simulink model "part_b"  (R2020b)
settings: Solver=VariableStepAuto  StartTime=0.0  StopTime=0.01  FixedStep=1e-9  RelTol=1e-3
libraries: powerlib x19, powerlib_meascontrol x1
settings Model: Creator=apurv  LastModifiedBy=apurv

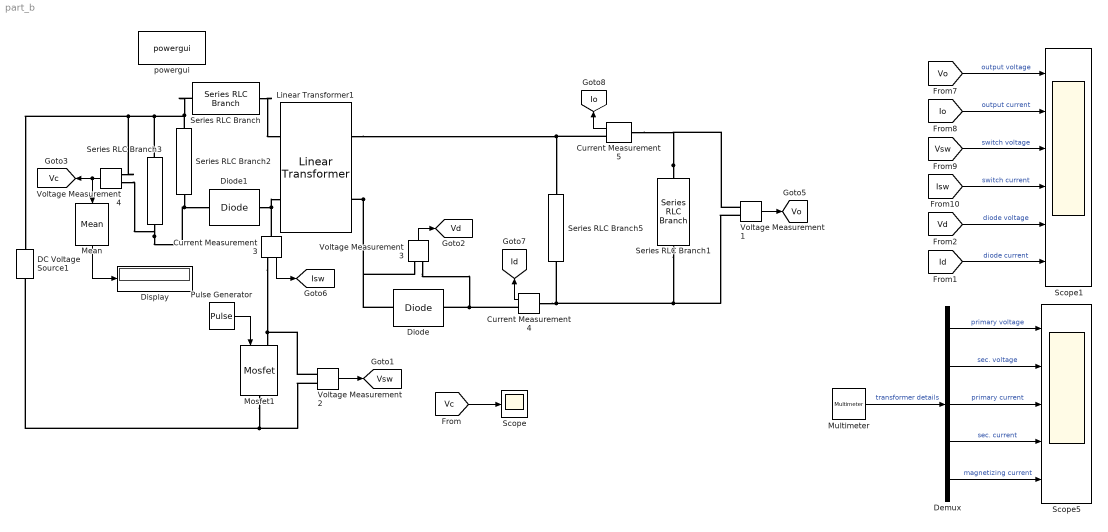
== system part_b ==
  Current Measurement3 : powerlib/Measurements/Current Measurement  PhasorSimulation=off  OutputType=Complex  PSBequivalent=0
  Current Measurement4 : powerlib/Measurements/Current Measurement  PhasorSimulation=off  OutputType=Complex  PSBequivalent=0
  Current Measurement5 : powerlib/Measurements/Current Measurement  PhasorSimulation=off  OutputType=Complex  PSBequivalent=0
  DC Voltage Source1 : powerlib/Electrical Sources/DC Voltage Source  Amplitude=24  Measurements=None
  Demux : Demux  Outputs=5
  Diode : powerlib/Power Electronics/Diode  Ron=1e-6  Lon=0  Vf=0  IC=0  UseSnubber=0  Rs=inf  Cs=0  Measurements=off
  Diode1 : powerlib/Power Electronics/Diode  Ron=1e-6  Lon=0  Vf=0  IC=0  UseSnubber=0  Rs=inf  Cs=0  Measurements=off
  Display : Display
  Linear Transformer1 : powerlib/Elements/Linear Transformer  UNITS=SI  NominalPower=[20 100000 ]  winding1=[30 0 0]  winding2=[10 0 0]  ThreeWindings=off  winding3=[3.15e+05 0.7938 0.084225]  RmLm=[1e12 250e-6]  Measurements=All voltages and currents  DataType=on
  Mean : powerlib_meascontrol/Measurements/Mean  Freq=100000  Vinit=0  Ts=0
  Mosfet1 : powerlib/Power Electronics/Mosfet  Ron=1e-6  Lon=0  Rd=1e-6  Vfd=0  IC=0  Rs=1e12  Cs=inf  Measurements=off
  Multimeter : powerlib/Measurements/Multimeter  PhasorSimulation=off  OutputType=Complex  sel=[1 2 3 4 6]  L=7  Gain=[1 1 1 1 1]  yselected={'Uw1: Linear Transformer1','Uw2: Linear Transformer1','Iw1: Linear Transformer1','Iw2: Linear Transformer1','Imag: Linear Transformer1'};  PSBOutputType=1  PSBequivalent=0  AxesSetting=[0,0.1,-100,100]  Display=0  SavedBlockNames=-11
  Pulse Generator : DiscretePulseGenerator  PulseType=Time based  Period=1/100000  PulseWidth=40
  Scope : Scope
  Scope1 : Scope  NumInputPorts=6
  Scope5 : Scope  NumInputPorts=5
  Series RLC Branch : powerlib/Elements/Series RLC Branch  LConnTagsString=__new0  RConnTagsString=__new0  BranchType=L  Resistance=1  Inductance=450e-9  SetiL0=off  InitialCurrent=0  Capacitance=1e-6  Setx0=off  InitialVoltage=0  Measurements=None
  Series RLC Branch1 : powerlib/Elements/Series RLC Branch  LConnTagsString=__new0  RConnTagsString=__new0  BranchType=R  Resistance=1  Inductance=1e-3  SetiL0=off  InitialCurrent=0  Capacitance=1e-6  Setx0=off  InitialVoltage=0  Measurements=None
  Series RLC Branch2 : powerlib/Elements/Series RLC Branch  LConnTagsString=__new0  RConnTagsString=__new0  BranchType=R  Resistance=5000  Inductance=1e-3  SetiL0=off  InitialCurrent=0  Capacitance=100e-6  Setx0=off  InitialVoltage=0  Measurements=None
  Series RLC Branch3 : powerlib/Elements/Series RLC Branch  LConnTagsString=__new0  RConnTagsString=__new0  BranchType=C  Resistance=0  Inductance=1e-3  SetiL0=off  InitialCurrent=0  Capacitance=10e-9  Setx0=off  InitialVoltage=0  Measurements=None
  Series RLC Branch5 : powerlib/Elements/Series RLC Branch  LConnTagsString=__new0  RConnTagsString=__new0  BranchType=C  Resistance=0  Inductance=1e-3  SetiL0=off  InitialCurrent=0  Capacitance=100e-6  Setx0=off  InitialVoltage=0  Measurements=None
  Voltage Measurement{1..4} (4 alike) : powerlib/Measurements/Voltage Measurement  PhasorSimulation=off  OutputType=Complex  PSBequivalent=0
  powergui : powerlib/powergui  Priority=1  SimulationMode=Discrete  SampleTime=1e-7  frequency=60  Iterations=50  frequencyindice=0  Pbase=100e6  ErrMax=1e-4  UnitsV=kV  UnitsW=MW  buscounter=0  FunctionMessages=off  echomessages=off  EnableUseOfTLC=off  CurrentSourceSwitches=off  DisableSnubberDevices=off  DisableRonSwitches=off  DisableVfSwitches=off  DisplayEquations=off  AutomaticDiscreteSolvers=off  SolverType=Tustin/Backward Euler (TBE)  Interpol=off  ExternalGateDelay=off  methode=off  Ts=100  x0status=blocks  SPID=on  SwTol=0  HookPort=off  NonlinearTolerance=1e-4  nMaxIteration=100  ContinueOnMaxIteration=off  RestoreLinks=warning  ResistiveCurrentMeasurement=off  Frange=[0:2:500]  Ylog=off  Xlog=on  ShowGrid=off  save=off  variable=ZData  structure=0  ZoomFFT=off  StartTime=0.0  cycles=1  DisplayStyle=1  fundamental=60  FreqAxis=off  MaxFrequency=1000  frequencyindicesteady=1  RmsSteady=1  display=off
  tag scope: Id=global, Io=global, Isw=global, Vc=global, Vd=global, Vo=global, Vsw=global
  wires:
  Demux/3 -> Scope5/3  "primary current"
  [Vo] -> Scope1/1  "output voltage"
  Multimeter/1 -> Demux/1  "transformer details"
  [Vd] -> Scope1/5  "diode voltage"
  Demux/5 -> Scope5/5  "magnetizing current"
  Demux/4 -> Scope5/4  "sec. current"
  Voltage Measurement2/1 -> [Vsw]
  [Io] -> Scope1/2  "output current"
  Voltage Measurement3/1 -> [Vd]
  [Id] -> Scope1/6  "diode current"
  Demux/1 -> Scope5/1  "primary voltage"
  [Isw] -> Scope1/4  "switch current"
  Current Measurement4/1 -> [Id]
  Current Measurement3/1 -> [Isw]
  [Vsw] -> Scope1/3  "switch voltage"
  Current Measurement5/1 -> [Io]
  Demux/2 -> Scope5/2  "sec. voltage"
  Voltage Measurement1/1 -> [Vo]
  Pulse Generator/1 -> Mosfet1/1
  Voltage Measurement4/1 -> Mean/1, [Vc]
  [Vc] -> Scope/1
  Mean/1 -> Display/1
  connections:
  Voltage Measurement2/LConn2 -- Mosfet1/RConn1 -- DC Voltage Source1/LConn1
  Voltage Measurement3/LConn2 -- Current Measurement4/RConn1 -- Diode/RConn1
  Linear Transformer1/RConn2 -- Diode/LConn1 -- Voltage Measurement3/LConn1
  Series RLC Branch1/LConn1 -- Current Measurement4/LConn1 -- Series RLC Branch5/LConn1 -- Voltage Measurement1/LConn1
  Mosfet1/LConn1 -- Current Measurement3/RConn1 -- Voltage Measurement2/LConn1
  Series RLC Branch1/RConn1 -- Voltage Measurement1/LConn2 -- Current Measurement5/LConn1
  Current Measurement5/RConn1 -- Linear Transformer1/RConn1 -- Series RLC Branch5/RConn1
  Current Measurement3/LConn1 -- Linear Transformer1/LConn2 -- Diode1/LConn1
  Series RLC Branch3/LConn1 -- Diode1/RConn1 -- Series RLC Branch2/LConn1 -- Voltage Measurement4/LConn1
  Series RLC Branch2/RConn1 -- Voltage Measurement4/LConn2 -- DC Voltage Source1/RConn1 -- Series RLC Branch3/RConn1 -- Series RLC Branch/LConn1
  Series RLC Branch/RConn1 -- Linear Transformer1/LConn1
